simulink model "TopLevel_Turbofan_DT_healthy"  (R2025a)
settings: Solver=ode15s  StartTime=0.0  StopTime=500  MaxStep=0.01  RelTol=1e-3
undefined symbols (not defined in the file or in its folder): BPR_design, Eff_Fan_v1, Eff_HPC_v1, Eff_hpt_map, Eff_HPT_v1, Eff_LPC_v1, Eff_LPT_v1, eta_hpc_map, eta_lpc_map, eta_lpt_map, Fan_eta_data, Fan_PR_data, flow_vec_fan, norm_flow_hpt, norm_speed_hpt, PDM_Data, PR_hpc_map, PR_lpc_map, PR_lpt_map, speed_vec_fan, speed_vec_hpc, speed_vec_lpc, speed_vec_lpt, Torque_hpt_map, Wc_hpc_bp, Wc_lpc_bp, Wc_lpt_bp
libraries: fl_lib x10, nesl_utility x10, sdl_lib x2
settings Model: Creator=ramch  LastModifiedBy=ramch
settings DataIOCC: SaveFormat=StructureWithTime

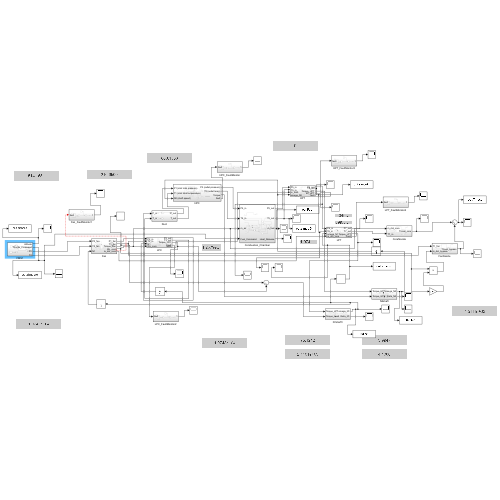
[thumbnail: Simulink's stored preview of the top-level diagram]
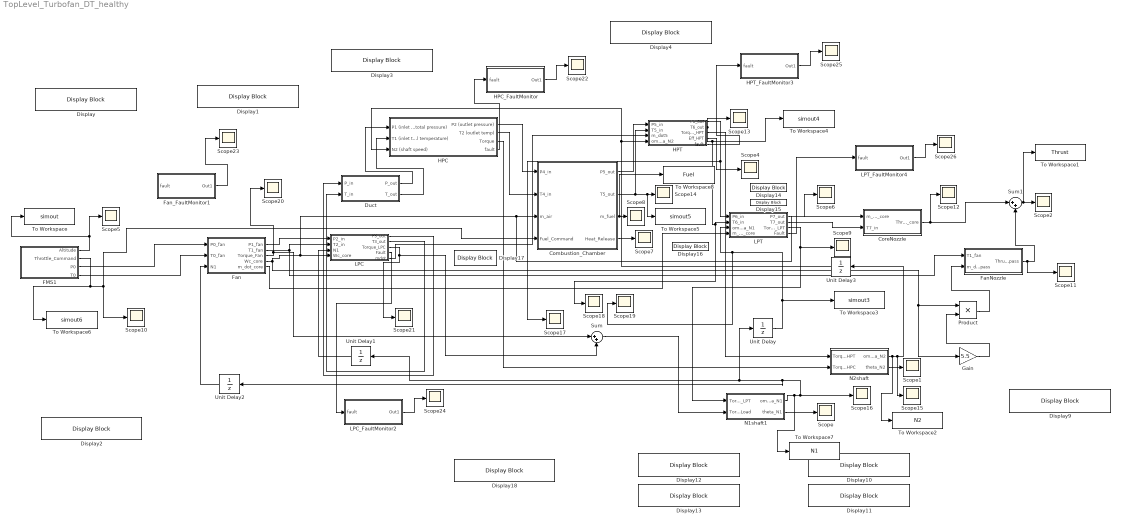
== system TopLevel_Turbofan_DT_healthy ==
  Combustion_Chamber : Subsystem
  CoreNozzle : Subsystem
  Display{,1..4,9..18} (15 alike) : DisplayBlock  LabelPosition=Hide  Transparency=1  GridColor=[0.502, 0.502, 0.502]
  Duct : Subsystem
  FMS1 : Subsystem
  Fan : Subsystem
  FanNozzle : Subsystem
  Fan_FaultMonitor1 : Subsystem
  Gain : Gain  Gain=5.5
  HPC : Subsystem
  HPC_FaultMonitor : Subsystem
  HPT : Subsystem
  HPT_FaultMonitor3 : Subsystem
  LPC : Subsystem
  LPC_FaultMonitor2 : Subsystem
  LPT : Subsystem
  LPT_FaultMonitor4 : Subsystem
  N1shaft1 : Subsystem
  N2shaft : Subsystem
  Product : Product
  Scope{,1..2,4..26} (26 alike) : Scope
      Scope settings: ActiveDisplayYMinimum=-1  ActiveDisplayYMaximum=1
      Scope1 settings: ActiveDisplayYMinimum=-1  ActiveDisplayYMaximum=1
      Scope10 settings: ActiveDisplayYMinimum=-0.45859345963387366  ActiveDisplayYMaximum=1.635778226221027  DataLoggingVariableName=ScopeData10
      Scope11 settings: ActiveDisplayYMinimum=-1  ActiveDisplayYMaximum=1  DataLoggingVariableName=ScopeData11
      Scope12 settings: ActiveDisplayYMinimum=-1  ActiveDisplayYMaximum=1  DataLoggingVariableName=ScopeData12
      Scope13 settings: ActiveDisplayYMinimum=-609.11434420859632  ActiveDisplayYMaximum=1781.0190470175871  DataLoggingVariableName=ScopeData13
      Scope14 settings: ActiveDisplayYMinimum=-1  ActiveDisplayYMaximum=1  DataLoggingVariableName=ScopeData14
      Scope15 settings: ActiveDisplayYMinimum=-1  ActiveDisplayYMaximum=1  DataLoggingVariableName=ScopeData15
      Scope16 settings: ActiveDisplayYMinimum=-4.3963021341582635  ActiveDisplayYMaximum=4.6281003390981308  DataLoggingVariableName=ScopeData16
      Scope17 settings: ActiveDisplayYMinimum=-2.2429279816897957E+23  ActiveDisplayYMaximum=2.0186351835208165E+24  DataLoggingVariableName=ScopeData17
      Scope18 settings: ActiveDisplayYMinimum=-513.71209028734575  ActiveDisplayYMaximum=1737.7811833983071  DataLoggingVariableName=ScopeData18
      Scope19 settings: ActiveDisplayYMinimum=-0.12499999999999997  ActiveDisplayYMaximum=1.125  DataLoggingVariableName=ScopeData19
      Scope2 settings: ActiveDisplayYMinimum=-1  ActiveDisplayYMaximum=1  DataLoggingVariableName=ScopeData2
      Scope20 settings: ActiveDisplayYMinimum=-3.6198875871994079E+21  ActiveDisplayYMaximum=5.5031192284267649E+20  DataLoggingVariableName=ScopeData20
      Scope21 settings: ActiveDisplayYMinimum=-0.23453341351778778  ActiveDisplayYMaximum=0.2421108240195578  DataLoggingVariableName=ScopeData21
      Scope22 settings: ActiveDisplayYMinimum=-609.11434420859632  ActiveDisplayYMaximum=1781.0190470175871  DataLoggingVariableName=ScopeData22
      Scope23 settings: ActiveDisplayYMinimum=-609.11434420859632  ActiveDisplayYMaximum=1781.0190470175871  DataLoggingVariableName=ScopeData23
      Scope24 settings: ActiveDisplayYMinimum=-609.11434420859632  ActiveDisplayYMaximum=1781.0190470175871  DataLoggingVariableName=ScopeData24
      Scope25 settings: ActiveDisplayYMinimum=-609.11434420859632  ActiveDisplayYMaximum=1781.0190470175871  DataLoggingVariableName=ScopeData25
      Scope26 settings: ActiveDisplayYMinimum=-609.11434420859632  ActiveDisplayYMaximum=1781.0190470175871  DataLoggingVariableName=ScopeData26
      Scope4 settings: ActiveDisplayYMinimum=-1.4197628335321743E+18  ActiveDisplayYMaximum=1.5775142594801933E+17  DataLoggingVariableName=ScopeData4
      Scope5 settings: ActiveDisplayYMinimum=-5201.9747686683695  ActiveDisplayYMaximum=12688.378863465885  DataLoggingVariableName=ScopeData5
      Scope6 settings: ActiveDisplayYMinimum=-1  ActiveDisplayYMaximum=1  DataLoggingVariableName=ScopeData6
      Scope7 settings: ActiveDisplayYMinimum=952444.62242727727  ActiveDisplayYMaximum=9.2631053030945715E+6  DataLoggingVariableName=ScopeData7
      Scope8 settings: ActiveDisplayYMinimum=-1  ActiveDisplayYMaximum=1  DataLoggingVariableName=ScopeData8
      Scope9 settings: ActiveDisplayYMinimum=-1  ActiveDisplayYMaximum=1  DataLoggingVariableName=ScopeData9
  Sum : Sum  Inputs=|++
  Sum1 : Sum  Inputs=|++
  To Workspace : ToWorkspace  VariableName=simout  SaveFormat=Timeseries  SampleTime=-1
  To Workspace1 : ToWorkspace  VariableName=Thrust  SaveFormat=Timeseries  SampleTime=-1
  To Workspace2 : ToWorkspace  VariableName=N2  SaveFormat=Timeseries  SampleTime=-1
  To Workspace3 : ToWorkspace  VariableName=simout3  SaveFormat=Timeseries  SampleTime=-1
  To Workspace4 : ToWorkspace  VariableName=simout4  SaveFormat=Timeseries  SampleTime=-1
  To Workspace5 : ToWorkspace  VariableName=simout5  SaveFormat=Timeseries  SampleTime=-1
  To Workspace6 : ToWorkspace  VariableName=simout6  SaveFormat=Timeseries  SampleTime=-1
  To Workspace7 : ToWorkspace  VariableName=N1  SaveFormat=Timeseries  SampleTime=-1
  To Workspace8 : ToWorkspace  VariableName=Fuel  SaveFormat=Timeseries  SampleTime=-1
  Unit Delay{,1..3} (4 alike) : UnitDelay  InitialCondition=1  SampleTime=-1  HasFrameUpgradeWarning=on
  wires:
  FMS1/3(P0) -> Fan/1(P0_fan)
  FMS1/4(T0) -> Fan/2(T0_fan)
  FMS1/2(Throttle_Command) -> To Workspace6/1, Combustion_Chamber/4(Fuel_Command), Scope10/1
  Fan/1(" P1_fan") -> LPC/1(P2_in)
  Fan/2(T1_fan) -> LPC/2(T2_in), FanNozzle/1(T1_fan)
  Fan/4(Wc_core) -> Gain/1, Product/1, CoreNozzle/1(m_dot_core), Combustion_Chamber/3(m_air), LPC/4(Wc_core)
  LPC/1(P3_out) -> Duct/1(P_in)
  Duct/1(P_out) -> HPC/1(P1 (inlet total pressure))
  Duct/2(T_out) -> HPC/2("T1 (inlet total temperature) ")
  HPC/1(P2 (outlet pressure)) -> Combustion_Chamber/1(P4_in)
  HPC/2(T2 (outlet temp)) -> Combustion_Chamber/2(T4_in)
  Combustion_Chamber/1(P5_out) -> HPT/1(P5_in)
  Combustion_Chamber/2(T5_out) -> To Workspace5/1, Scope14/1, HPT/2(T5_in)
  HPT/1(P6_out) -> LPT/1(P6_in), Scope17/1
  HPT/2(T6_out) -> To Workspace4/1, Scope18/1, LPT/2(T6_in), Scope13/1
  LPT/3(Torque_LPT) -> N1shaft1/1(Torque_LPT), Scope9/1
  Sum/1 -> N1shaft1/2(Torque_Load)
  LPC/3(Torque_LPC) -> Scope21/1, Sum/2
  Fan/3(Torque_Fan) -> Scope20/1, Sum/1
  HPC/3(Torque) -> N2shaft/2(Torque_HPC)
  HPT/3(Torque_HPT) -> N2shaft/1(Torque_HPT)
  N2shaft/1(omega_N2) -> To Workspace2/1, Scope15/1, Unit Delay3/1
  LPT/2(T7_out) -> CoreNozzle/2(T7_in)
  Product/1 -> FanNozzle/2(m_dot_bypass)
  Gain/1 -> Product/2
  FanNozzle/1(Thrust_bypass) -> Scope11/1, Sum1/2
  CoreNozzle/1(Thrust_core) -> Scope12/1, Sum1/1
  Sum1/1 -> To Workspace1/1, Scope2/1
  N2shaft/2(theta_N2) -> Scope1/1
  LPC/2(T3_out) -> Duct/2(T_in)
  FMS1/1(Altitude) -> To Workspace/1, Scope5/1
  HPT/4(Eff_HPT) -> Scope4/1
  LPT/1(P7_out) -> Scope6/1
  Combustion_Chamber/3(m_fuel) -> To Workspace8/1, Scope8/1
  Combustion_Chamber/4(Heat_Release) -> Scope7/1
  N1shaft1/2(theta_N1) -> Scope/1
  N1shaft1/1(omega_N1) -> To Workspace7/1, Unit Delay/1, Unit Delay1/1, Unit Delay2/1, Scope16/1
  Unit Delay/1 -> Scope19/1, LPT/3(omega_N1), To Workspace3/1
  Unit Delay2/1 -> Fan/3(N1)
  Unit Delay1/1 -> LPC/3(N1)
  HPC_FaultMonitor/1(Out1) -> Scope22/1
  HPC/4(fault) -> HPC_FaultMonitor/1(fault)
  Fan_FaultMonitor1/1(Out1) -> Scope23/1
  LPC_FaultMonitor2/1(Out1) -> Scope24/1
  HPT_FaultMonitor3/1(Out1) -> Scope25/1
  LPT_FaultMonitor4/1(Out1) -> Scope26/1
  ? -> Fan_FaultMonitor1/1(fault)
  LPC/4(Fault) -> LPC_FaultMonitor2/1(fault)
  HPT/5(fault) -> HPT_FaultMonitor3/1(fault)
  LPT/4(Fault) -> LPT_FaultMonitor4/1(fault)
  Unit Delay3/1 -> HPT/4(omega_N2), HPC/3(N2 (shaft speed))
  LPC/5(mdot) -> HPT/3(m_dot5)
  Fan/5(m_dot_core) -> LPT/4(m_dot_core)

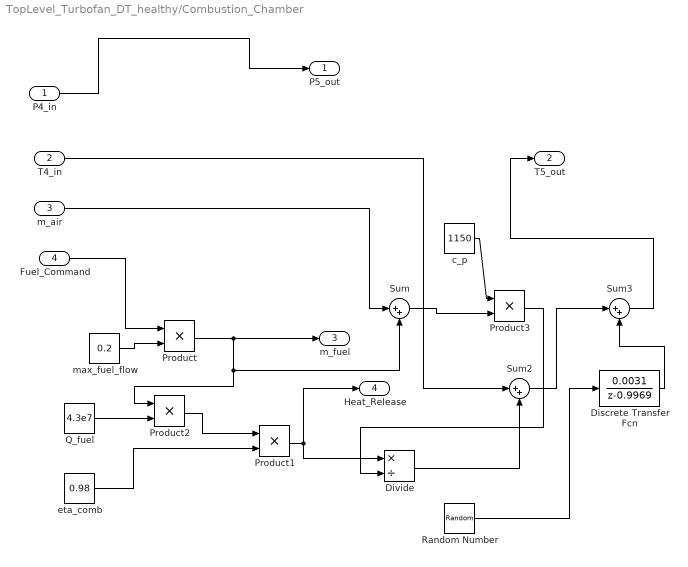
== system TopLevel_Turbofan_DT_healthy/Combustion_Chamber ==
  P4_in : Inport
  T4_in : Inport  Port=2
  m_air : Inport  Port=3
  Fuel_Command : Inport  Port=4
  Discrete Transfer Fcn : DiscreteTransferFcn  Numerator=0.0031  Denominator=1 -0.9969  InitialStates=0.001
  Divide : Product  Inputs=*/
  Product{,1..3} (4 alike) : Product
  Q_fuel : Constant  Value=4.3e7
  Random Number : RandomNumber  Variance=0.5  SampleTime=0.001
  Sum : Sum  Inputs=|++
  Sum2 : Sum  Inputs=|++
  Sum3 : Sum  Inputs=|++
  c_p : Constant  Value=1150
  eta_comb : Constant  Value=0.98
  max_fuel_flow : Constant  Value=0.2
  P5_out : Outport
  T5_out : Outport  Port=2
  m_fuel : Outport  Port=3
  Heat_Release : Outport  Port=4
  wires:
  Discrete Transfer Fcn/1 -> Sum3/2
  Sum2/1 -> Sum3/1
  Sum3/1 -> T5_out/1
  Random Number/1 -> Discrete Transfer Fcn/1
  Divide/1 -> Sum2/2
  T4_in/1 -> Sum2/1
  Product3/1 -> Divide/2
  c_p/1 -> Product3/1
  Sum/1 -> Product3/2
  P4_in/1 -> P5_out/1
  m_air/1 -> Sum/1
  Product2/1 -> Product1/1
  Product/1 -> m_fuel/1, Sum/2, Product2/1
  Product1/1 -> Divide/1, Heat_Release/1
  eta_comb/1 -> Product1/2
  Q_fuel/1 -> Product2/2
  max_fuel_flow/1 -> Product/2
  Fuel_Command/1 -> Product/1

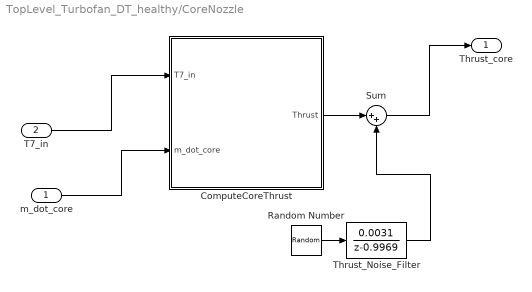
== system TopLevel_Turbofan_DT_healthy/CoreNozzle ==
  m_dot_core : Inport
  T7_in : Inport  Port=2
  ComputeCoreThrust : MATLAB Function  TreatAsAtomicUnit=on
  Random Number : RandomNumber  Variance=500  SampleTime=0.001
  Sum : Sum  Inputs=|++
  Thrust_Noise_Filter : DiscreteTransferFcn  Numerator=0.0031  Denominator=1 -0.9969  InitialStates=0.001
  Thrust_core : Outport
  wires:
  Sum/1 -> Thrust_core/1
  T7_in/1 -> ComputeCoreThrust/1(T7_in)
  Random Number/1 -> Thrust_Noise_Filter/1
  m_dot_core/1 -> ComputeCoreThrust/2(m_dot_core)
  ComputeCoreThrust/1(Thrust) -> Sum/1
  Thrust_Noise_Filter/1 -> Sum/2

== system TopLevel_Turbofan_DT_healthy/Duct ==
  P_in : Inport
  T_in : Inport  Port=2
  Gain : Gain  Gain=0.98
  P_out : Outport
  T_out : Outport  Port=2
  wires:
  Gain/1 -> P_out/1
  T_in/1 -> T_out/1
  P_in/1 -> Gain/1

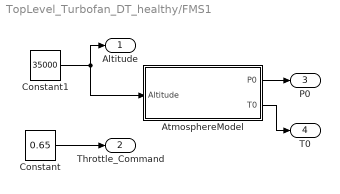
== system TopLevel_Turbofan_DT_healthy/FMS1 ==
  AtmosphereModel : MATLAB Function  TreatAsAtomicUnit=on
  Constant : Constant  Value=0.65
  Constant1 : Constant  Value=35000
  Altitude : Outport
  Throttle_Command : Outport  Port=2
  P0 : Outport  Port=3
  T0 : Outport  Port=4
  wires:
  AtmosphereModel/1(P0) -> P0/1
  AtmosphereModel/2(T0) -> T0/1
  Constant1/1 -> AtmosphereModel/1(Altitude), Altitude/1
  Constant/1 -> Throttle_Command/1

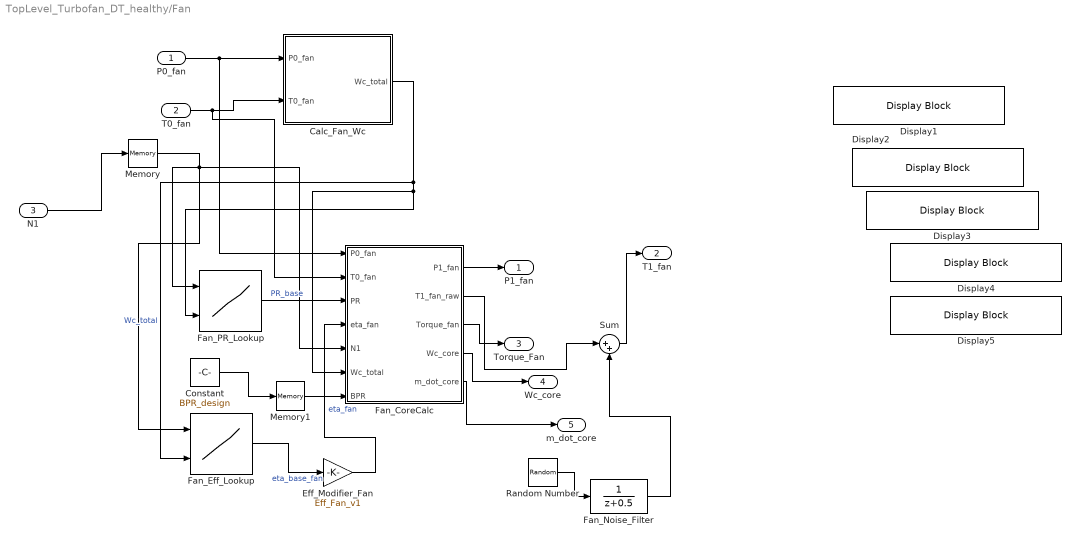
== system TopLevel_Turbofan_DT_healthy/Fan ==
  P0_fan : Inport
  T0_fan : Inport  Port=2
  N1 : Inport  Port=3
  Calc_Fan_Wc : MATLAB Function  TreatAsAtomicUnit=on
  Constant : Constant  Value=BPR_design
  Display{1..5} (5 alike) : DisplayBlock  LabelPosition=Hide  Transparency=1  GridColor=[0.502, 0.502, 0.502]
  Eff_Modifier_Fan : Gain  Gain=Eff_Fan_v1
  Fan_CoreCalc : MATLAB Function  TreatAsAtomicUnit=on
  Fan_Eff_Lookup : Lookup_n-D  BreakpointsForDimension1=speed_vec_fan  BreakpointsForDimension2=flow_vec_fan  Table=Fan_eta_data  ExtrapMethod=Clip  InternalRulePriority=Speed  RndMeth=Simplest
      settings: InputPortMap=u0,u1
  Fan_Noise_Filter : DiscreteTransferFcn
  Fan_PR_Lookup : Lookup_n-D  BreakpointsForDimension1=speed_vec_fan  BreakpointsForDimension2=flow_vec_fan  Table=Fan_PR_data  ExtrapMethod=Clip  InternalRulePriority=Speed  RndMeth=Simplest
      settings: InputPortMap=u0,u1
  Memory : Memory
  Memory1 : Memory
  Random Number : RandomNumber  Variance=(0.5)  SampleTime=0.001
  Sum : Sum  Inputs=|++
  " P1_fan" : Outport
  T1_fan : Outport  Port=2
  Torque_Fan : Outport  Port=3
  Wc_core : Outport  Port=4
  m_dot_core : Outport  Port=5
  wires:
  Random Number/1 -> Fan_Noise_Filter/1
  Fan_Noise_Filter/1 -> Sum/2
  Fan_CoreCalc/2(T1_fan_raw) -> Sum/1
  Sum/1 -> T1_fan/1
  Fan_CoreCalc/1(P1_fan) -> " P1_fan"/1
  Fan_CoreCalc/3(Torque_fan) -> Torque_Fan/1
  Fan_CoreCalc/4(Wc_core) -> Wc_core/1
  Fan_PR_Lookup/1 -> Fan_CoreCalc/3(PR)  "PR_base"
  Eff_Modifier_Fan/1 -> Fan_CoreCalc/4(eta_fan)  "eta_fan"
  Fan_Eff_Lookup/1 -> Eff_Modifier_Fan/1  "eta_base_fan"
  Calc_Fan_Wc/1(Wc_total) -> Fan_Eff_Lookup/2, Fan_PR_Lookup/2, Fan_CoreCalc/6(Wc_total)  "Wc_total"
  T0_fan/1 -> Calc_Fan_Wc/2(T0_fan), Fan_CoreCalc/2(T0_fan)
  P0_fan/1 -> Calc_Fan_Wc/1(P0_fan), Fan_CoreCalc/1(P0_fan)
  Memory1/1 -> Fan_CoreCalc/7(BPR)
  Memory/1 -> Fan_Eff_Lookup/1, Fan_PR_Lookup/1, Fan_CoreCalc/5(N1)
  Constant/1 -> Memory1/1
  N1/1 -> Memory/1
  Fan_CoreCalc/5(m_dot_core) -> m_dot_core/1

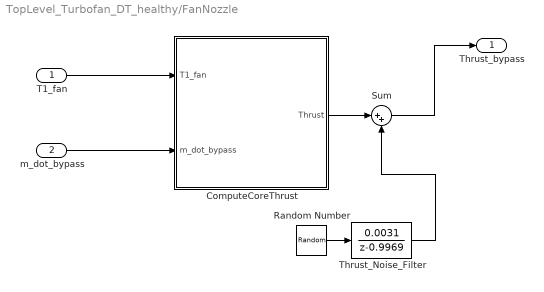
== system TopLevel_Turbofan_DT_healthy/FanNozzle ==
  T1_fan : Inport
  m_dot_bypass : Inport  Port=2
  ComputeCoreThrust : MATLAB Function  TreatAsAtomicUnit=on
  Random Number : RandomNumber  Variance=200  SampleTime=0.001
  Sum : Sum  Inputs=|++
  Thrust_Noise_Filter : DiscreteTransferFcn  Numerator=0.0031  Denominator=1 -0.9969  InitialStates=0.001
  Thrust_bypass : Outport
  wires:
  T1_fan/1 -> ComputeCoreThrust/1(T1_fan)
  Random Number/1 -> Thrust_Noise_Filter/1
  Sum/1 -> Thrust_bypass/1
  Thrust_Noise_Filter/1 -> Sum/2
  ComputeCoreThrust/1(Thrust) -> Sum/1
  m_dot_bypass/1 -> ComputeCoreThrust/2(m_dot_bypass)

== system TopLevel_Turbofan_DT_healthy/Fan_FaultMonitor1 ==
  fault : Inport
  Constant : Constant  Value=0.95
  Constant1 : Constant  Value=0.05
  Relational Operator : RelationalOperator  Operator=>  OutDataTypeStr=boolean  RndMeth=Simplest  InputSameDT=off
  Subtract : Sum  Inputs=+-
  Out1 : Outport
  wires:
  Constant/1 -> Subtract/1
  fault/1 -> Subtract/2
  Subtract/1 -> Relational Operator/2
  Constant1/1 -> Relational Operator/1
  Relational Operator/1 -> Out1/1

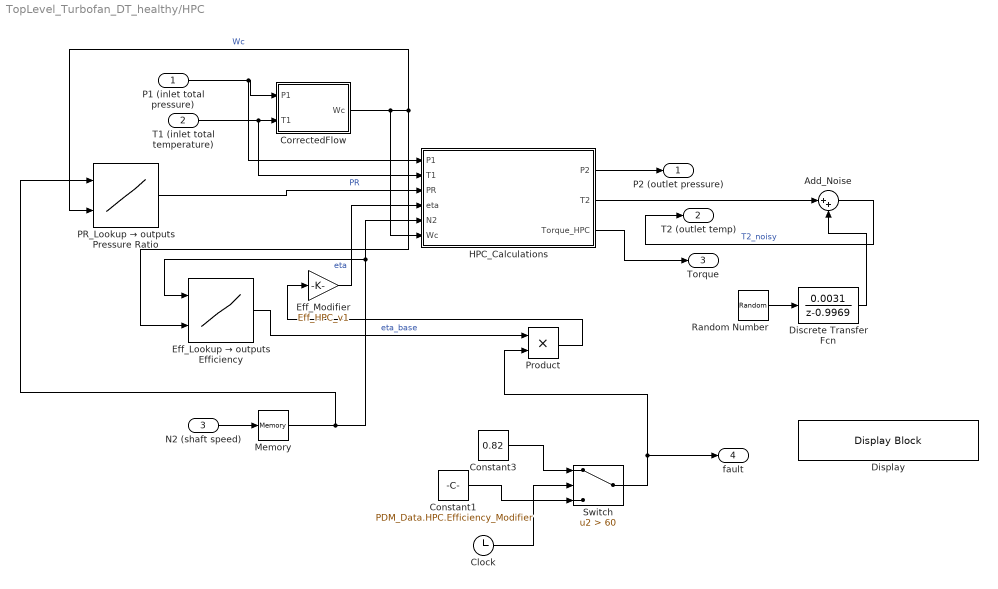
== system TopLevel_Turbofan_DT_healthy/HPC ==
  P1 (inlet total pressure) : Inport
  "T1 (inlet total temperature) " : Inport  Port=2
  N2 (shaft speed) : Inport  Port=3
  Add_Noise : Sum  Inputs=|++
  Clock : Clock
  Constant1 : Constant  Value=PDM_Data.HPC.Efficiency_Modifier
  Constant3 : Constant  Value=0.82
  CorrectedFlow : MATLAB Function  TreatAsAtomicUnit=on
  Discrete Transfer Fcn : DiscreteTransferFcn  Numerator=0.0031  Denominator=1 -0.9969  InitialStates=0.001
  Display : DisplayBlock  LabelPosition=Hide  Transparency=1  GridColor=[0.502, 0.502, 0.502]
  Eff_Lookup → outputs Efficiency : Lookup_n-D  BreakpointsForDimension1=speed_vec_hpc  BreakpointsForDimension2=Wc_hpc_bp  Table=eta_hpc_map  InternalRulePriority=Speed  RndMeth=Simplest
      settings: InputPortMap=u0,u1
  Eff_Modifier : Gain  Gain=Eff_HPC_v1
  HPC_Calculations : MATLAB Function  TreatAsAtomicUnit=on
  Memory : Memory
  PR_Lookup → outputs Pressure Ratio : Lookup_n-D  BreakpointsForDimension1=speed_vec_hpc  BreakpointsForDimension2=Wc_hpc_bp  Table=PR_hpc_map  InternalRulePriority=Speed  RndMeth=Simplest
      settings: InputPortMap=u0,u1
  Product : Product
  Random Number : RandomNumber  Variance=(0.5)  SampleTime=0.001
  Switch : Switch  Criteria=u2 > Threshold  Threshold=60  SaturateOnIntegerOverflow=off  InputSameDT=off
  P2 (outlet pressure) : Outport
  T2 (outlet temp) : Outport  Port=2
  Torque : Outport  Port=3
  fault : Outport  Port=4
  wires:
  Random Number/1 -> Discrete Transfer Fcn/1
  Discrete Transfer Fcn/1 -> Add_Noise/2
  Add_Noise/1 -> T2 (outlet temp)/1  "T2_noisy"
  Eff_Modifier/1 -> HPC_Calculations/4(eta)  "eta"
  CorrectedFlow/1(Wc) -> Eff_Lookup → outputs Efficiency/2, PR_Lookup → outputs Pressure Ratio/2, HPC_Calculations/6(Wc)  "Wc"
  "T1 (inlet total temperature) "/1 -> CorrectedFlow/2(T1), HPC_Calculations/2(T1)
  P1 (inlet total pressure)/1 -> CorrectedFlow/1(P1), HPC_Calculations/1(P1)
  N2 (shaft speed)/1 -> Memory/1
  Eff_Lookup → outputs Efficiency/1 -> Product/1  "eta_base"
  PR_Lookup → outputs Pressure Ratio/1 -> HPC_Calculations/3(PR)  "PR"
  HPC_Calculations/3(Torque_HPC) -> Torque/1
  HPC_Calculations/2(T2) -> Add_Noise/1
  HPC_Calculations/1(P2) -> P2 (outlet pressure)/1
  Memory/1 -> HPC_Calculations/5(N2), Eff_Lookup → outputs Efficiency/1, PR_Lookup → outputs Pressure Ratio/1
  Product/1 -> Eff_Modifier/1
  Constant3/1 -> Switch/1
  Switch/1 -> Product/2, fault/1
  Clock/1 -> Switch/2
  Constant1/1 -> Switch/3

== system TopLevel_Turbofan_DT_healthy/HPC_FaultMonitor ==
  fault : Inport
  Constant : Constant  Value=0.92
  Constant1 : Constant  Value=0.05
  Relational Operator : RelationalOperator  Operator=>  OutDataTypeStr=boolean  RndMeth=Simplest  InputSameDT=off
  Subtract : Sum  Inputs=+-
  Out1 : Outport
  wires:
  Constant/1 -> Subtract/1
  fault/1 -> Subtract/2
  Subtract/1 -> Relational Operator/2
  Constant1/1 -> Relational Operator/1
  Relational Operator/1 -> Out1/1

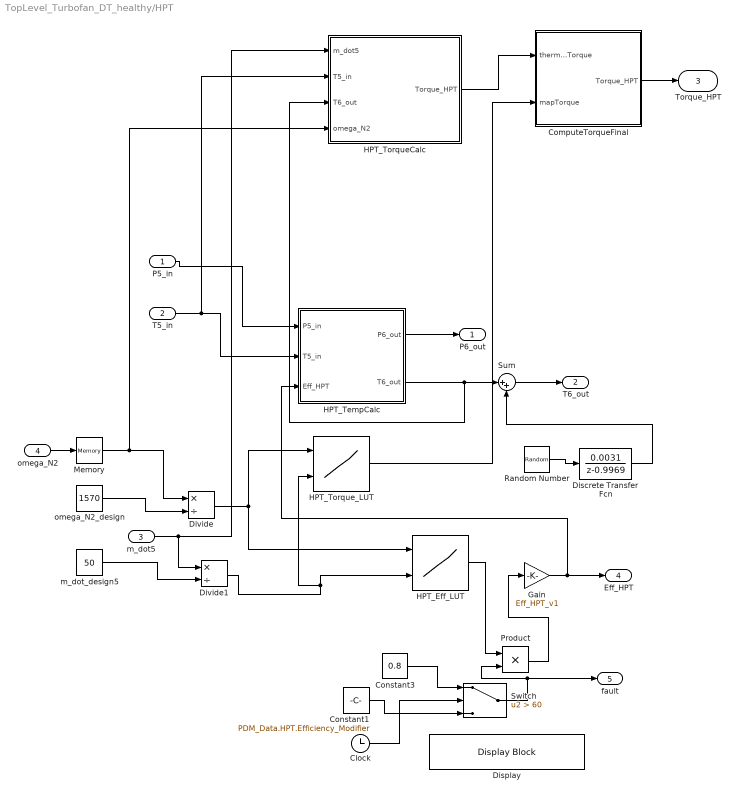
== system TopLevel_Turbofan_DT_healthy/HPT ==
  P5_in : Inport
  T5_in : Inport  Port=2
  m_dot5 : Inport  Port=3
  omega_N2 : Inport  Port=4
  Clock : Clock
  ComputeTorqueFinal : MATLAB Function  TreatAsAtomicUnit=on
  Constant1 : Constant  Value=PDM_Data.HPT.Efficiency_Modifier
  Constant3 : Constant  Value=0.8
  Discrete Transfer Fcn : DiscreteTransferFcn  Numerator=0.0031  Denominator=1 -0.9969  InitialStates=0.001
  Display : DisplayBlock  LabelPosition=Hide  Transparency=1  GridColor=[0.502, 0.502, 0.502]
  Divide : Product  Inputs=*/
  Divide1 : Product  Inputs=*/
  Gain : Gain  Gain=Eff_HPT_v1
  HPT_Eff_LUT : Lookup_n-D  BreakpointsForDimension1=norm_speed_hpt  BreakpointsForDimension2=norm_flow_hpt  Table=Eff_hpt_map  InternalRulePriority=Speed  RndMeth=Simplest
      settings: InputPortMap=u0,u1
  HPT_TempCalc : MATLAB Function  TreatAsAtomicUnit=on
  HPT_TorqueCalc : MATLAB Function  TreatAsAtomicUnit=on
  HPT_Torque_LUT : Lookup_n-D  BreakpointsForDimension1=norm_speed_hpt  BreakpointsForDimension2=norm_flow_hpt  Table=Torque_hpt_map  InternalRulePriority=Speed  RndMeth=Simplest
      settings: InputPortMap=u0,u1
  Memory : Memory
  Product : Product
  Random Number : RandomNumber  Variance=0.5  SampleTime=0.1
  Sum : Sum  Inputs=|++
  Switch : Switch  Criteria=u2 > Threshold  Threshold=60  SaturateOnIntegerOverflow=off  InputSameDT=off
  m_dot_design5 : Constant  Value=50
  omega_N2_design : Constant  Value=1570
  P6_out : Outport
  T6_out : Outport  Port=2
  Torque_HPT : Outport  Port=3
  Eff_HPT : Outport  Port=4
  fault : Outport  Port=5
  wires:
  HPT_Torque_LUT/1 -> ComputeTorqueFinal/2(mapTorque)
  HPT_TorqueCalc/1(Torque_HPT) -> ComputeTorqueFinal/1(thermoTorque)
  ComputeTorqueFinal/1(Torque_HPT) -> Torque_HPT/1
  Random Number/1 -> Discrete Transfer Fcn/1
  Sum/1 -> T6_out/1
  Discrete Transfer Fcn/1 -> Sum/2
  HPT_TempCalc/2(T6_out) -> Sum/1, HPT_TorqueCalc/3(T6_out)
  HPT_TempCalc/1(P6_out) -> P6_out/1
  T5_in/1 -> HPT_TempCalc/2(T5_in), HPT_TorqueCalc/2(T5_in)
  Gain/1 -> Eff_HPT/1, HPT_TempCalc/3(Eff_HPT)
  HPT_Eff_LUT/1 -> Product/1
  P5_in/1 -> HPT_TempCalc/1(P5_in)
  Divide1/1 -> HPT_Eff_LUT/2, HPT_Torque_LUT/2
  Divide/1 -> HPT_Torque_LUT/1, HPT_Eff_LUT/1
  omega_N2/1 -> Memory/1
  omega_N2_design/1 -> Divide/2
  m_dot5/1 -> Divide1/1, HPT_TorqueCalc/1(m_dot5)
  m_dot_design5/1 -> Divide1/2
  Memory/1 -> Divide/1, HPT_TorqueCalc/4(omega_N2)
  Product/1 -> Gain/1
  Constant3/1 -> Switch/1
  Switch/1 -> fault/1, Product/2
  Clock/1 -> Switch/2
  Constant1/1 -> Switch/3

== system TopLevel_Turbofan_DT_healthy/HPT_FaultMonitor3 ==
  fault : Inport
  Constant : Constant  Value=0.97
  Constant1 : Constant  Value=0.05
  Relational Operator : RelationalOperator  Operator=>  OutDataTypeStr=boolean  RndMeth=Simplest  InputSameDT=off
  Subtract : Sum  Inputs=+-
  Out1 : Outport
  wires:
  Constant/1 -> Subtract/1
  fault/1 -> Subtract/2
  Subtract/1 -> Relational Operator/2
  Constant1/1 -> Relational Operator/1
  Relational Operator/1 -> Out1/1

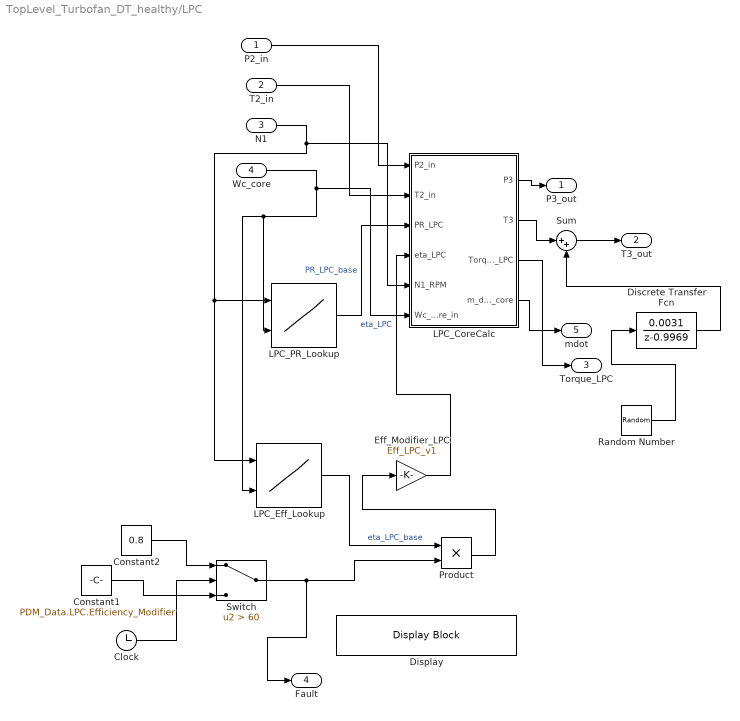
== system TopLevel_Turbofan_DT_healthy/LPC ==
  P2_in : Inport
  T2_in : Inport  Port=2
  N1 : Inport  Port=3
  Wc_core : Inport  Port=4
  Clock : Clock
  Constant1 : Constant  Value=PDM_Data.LPC.Efficiency_Modifier
  Constant2 : Constant  Value=0.8
  Discrete Transfer Fcn : DiscreteTransferFcn  Numerator=0.0031  Denominator=1 -0.9969  InitialStates=0.001
  Display : DisplayBlock  LabelPosition=Hide  Transparency=1  GridColor=[0.502, 0.502, 0.502]
  Eff_Modifier_LPC : Gain  Gain=Eff_LPC_v1
  LPC_CoreCalc : MATLAB Function  TreatAsAtomicUnit=on
  LPC_Eff_Lookup : Lookup_n-D  BreakpointsForDimension1=speed_vec_lpc  BreakpointsForDimension2=Wc_lpc_bp  Table=eta_lpc_map  ExtrapMethod=Clip  InternalRulePriority=Speed  RndMeth=Simplest
      settings: InputPortMap=u0,u1
  LPC_PR_Lookup : Lookup_n-D  BreakpointsForDimension1=speed_vec_lpc  BreakpointsForDimension2=Wc_lpc_bp  Table=PR_lpc_map  ExtrapMethod=Clip  InternalRulePriority=Speed  RndMeth=Simplest
      settings: InputPortMap=u0,u1
  Product : Product
  Random Number : RandomNumber  Variance=(0.5)  SampleTime=0.001
  Sum : Sum  Inputs=|++
  Switch : Switch  Criteria=u2 > Threshold  Threshold=60  SaturateOnIntegerOverflow=off  InputSameDT=off
  P3_out : Outport
  T3_out : Outport  Port=2
  Torque_LPC : Outport  Port=3
  Fault : Outport  Port=4
  mdot : Outport  Port=5
  wires:
  Discrete Transfer Fcn/1 -> Sum/2
  Random Number/1 -> Discrete Transfer Fcn/1
  Sum/1 -> T3_out/1
  LPC_CoreCalc/2(T3) -> Sum/1
  LPC_CoreCalc/3(Torque_LPC) -> Torque_LPC/1
  LPC_CoreCalc/1(P3) -> P3_out/1
  Eff_Modifier_LPC/1 -> LPC_CoreCalc/4(eta_LPC)  "eta_LPC"
  LPC_PR_Lookup/1 -> LPC_CoreCalc/3(PR_LPC)  "PR_LPC_base"
  T2_in/1 -> LPC_CoreCalc/2(T2_in)
  P2_in/1 -> LPC_CoreCalc/1(P2_in)
  LPC_Eff_Lookup/1 -> Product/1  "eta_LPC_base"
  Wc_core/1 -> LPC_PR_Lookup/2, LPC_Eff_Lookup/2, LPC_CoreCalc/6(Wc_core_in)
  N1/1 -> LPC_PR_Lookup/1, LPC_Eff_Lookup/1, LPC_CoreCalc/5(N1_RPM)
  Product/1 -> Eff_Modifier_LPC/1
  Constant2/1 -> Switch/1
  Switch/1 -> Fault/1, Product/2
  LPC_CoreCalc/4(m_dot_core) -> mdot/1
  Clock/1 -> Switch/2
  Constant1/1 -> Switch/3

== system TopLevel_Turbofan_DT_healthy/LPC_FaultMonitor2 ==
  fault : Inport
  Constant : Constant  Value=0.9
  Constant1 : Constant  Value=0.05
  Relational Operator : RelationalOperator  Operator=>  OutDataTypeStr=boolean  RndMeth=Simplest  InputSameDT=off
  Subtract : Sum  Inputs=+-
  Out1 : Outport
  wires:
  Constant/1 -> Subtract/1
  fault/1 -> Subtract/2
  Subtract/1 -> Relational Operator/2
  Constant1/1 -> Relational Operator/1
  Relational Operator/1 -> Out1/1

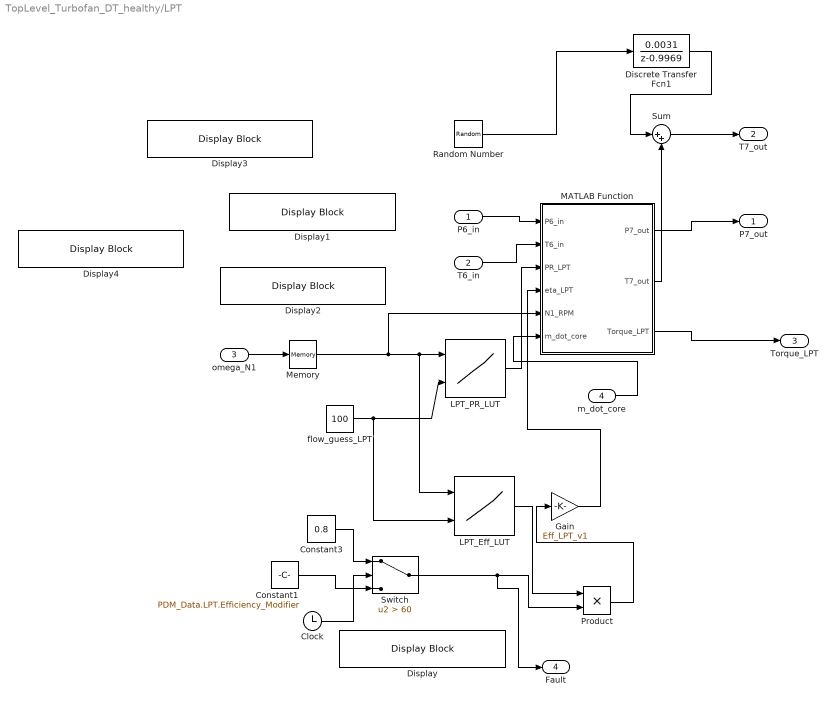
== system TopLevel_Turbofan_DT_healthy/LPT ==
  P6_in : Inport
  T6_in : Inport  Port=2
  omega_N1 : Inport  Port=3
  m_dot_core : Inport  Port=4
  Clock : Clock
  Constant1 : Constant  Value=PDM_Data.LPT.Efficiency_Modifier
  Constant3 : Constant  Value=0.8
  Discrete Transfer Fcn1 : DiscreteTransferFcn  Numerator=0.0031  Denominator=1 -0.9969  InitialStates=0.001
  Display{,1..4} (5 alike) : DisplayBlock  LabelPosition=Hide  Transparency=1  GridColor=[0.502, 0.502, 0.502]
  Gain : Gain  Gain=Eff_LPT_v1
  LPT_Eff_LUT : Lookup_n-D  BreakpointsForDimension1=speed_vec_lpt  BreakpointsForDimension2=Wc_lpt_bp  Table=eta_lpt_map  ExtrapMethod=Clip  InternalRulePriority=Speed  RndMeth=Simplest
      settings: InputPortMap=u0,u1
  LPT_PR_LUT : Lookup_n-D  BreakpointsForDimension1=speed_vec_lpt  BreakpointsForDimension2=Wc_lpt_bp  Table=PR_lpt_map  ExtrapMethod=Clip  InternalRulePriority=Speed  RndMeth=Simplest
      settings: InputPortMap=u0,u1
  MATLAB Function : MATLAB Function  TreatAsAtomicUnit=on
  Memory : Memory
  Product : Product
  Random Number : RandomNumber  Variance=0.5  SampleTime=0.001
  Sum : Sum  Inputs=|++
  Switch : Switch  Criteria=u2 > Threshold  Threshold=60  SaturateOnIntegerOverflow=off  InputSameDT=off
  flow_guess_LPT : Constant  Value=100
  P7_out : Outport
  T7_out : Outport  Port=2
  Torque_LPT : Outport  Port=3
  Fault : Outport  Port=4
  wires:
  MATLAB Function/2(T7_out) -> Sum/2
  Gain/1 -> MATLAB Function/4(eta_LPT)
  LPT_Eff_LUT/1 -> Product/1
  MATLAB Function/1(P7_out) -> P7_out/1
  MATLAB Function/3(Torque_LPT) -> Torque_LPT/1
  flow_guess_LPT/1 -> LPT_Eff_LUT/2, LPT_PR_LUT/2
  omega_N1/1 -> Memory/1
  T6_in/1 -> MATLAB Function/2(T6_in)
  Sum/1 -> T7_out/1
  Discrete Transfer Fcn1/1 -> Sum/1
  Random Number/1 -> Discrete Transfer Fcn1/1
  LPT_PR_LUT/1 -> MATLAB Function/3(PR_LPT)
  P6_in/1 -> MATLAB Function/1(P6_in)
  Memory/1 -> LPT_PR_LUT/1, LPT_Eff_LUT/1, MATLAB Function/5(N1_RPM)
  Product/1 -> Gain/1
  Constant3/1 -> Switch/1
  Switch/1 -> Fault/1, Product/2
  Constant1/1 -> Switch/3
  Clock/1 -> Switch/2
  m_dot_core/1 -> MATLAB Function/6(m_dot_core)

== system TopLevel_Turbofan_DT_healthy/LPT_FaultMonitor4 ==
  fault : Inport
  Constant : Constant  Value=0.96
  Constant1 : Constant  Value=0.05
  Relational Operator : RelationalOperator  Operator=>  OutDataTypeStr=boolean  RndMeth=Simplest  InputSameDT=off
  Subtract : Sum  Inputs=+-
  Out1 : Outport
  wires:
  Constant/1 -> Subtract/1
  fault/1 -> Subtract/2
  Subtract/1 -> Relational Operator/2
  Constant1/1 -> Relational Operator/1
  Relational Operator/1 -> Out1/1

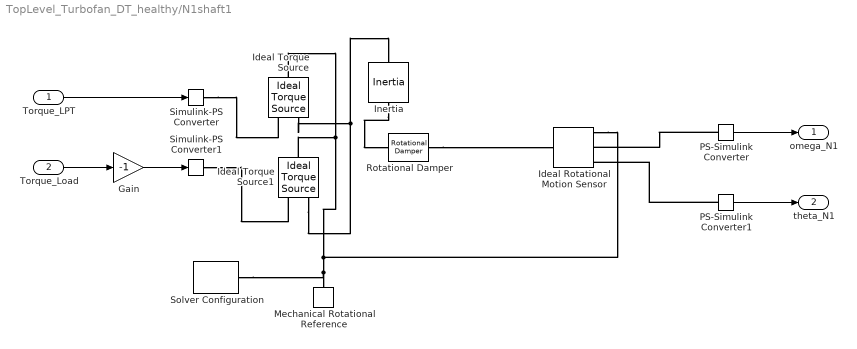
== system TopLevel_Turbofan_DT_healthy/N1shaft1 ==
  Torque_LPT : Inport
  Torque_Load : Inport  Port=2
  Gain : Gain  Gain=-1
  Ideal Rotational Motion Sensor : fl_lib/Mechanical/Mechanical Sensors/Ideal Rotational Motion Sensor  reference=foundation.enum.MeasurementReference.difference  acceleration_port=false  velocity_port=true  position_port=true  wrap_angle=false  offset=0 rad
  Ideal Torque Source : fl_lib/Mechanical/Mechanical Sources/Ideal Torque Source
  Ideal Torque Source1 : fl_lib/Mechanical/Mechanical Sources/Ideal Torque Source
  Inertia : fl_lib/Mechanical/Rotational Elements/Inertia  inertia=100 kg*m^2  num_ports=foundation.enum.numPorts2.two  w_specify=off  w_priority=High  w=52.36 rad/s  w_nominal_specify=off  w_nominal_value=1  w_nominal_unit=rad/s  t_specify=off  t_priority=None  t=0 N*m  t_nominal_specify=off  t_nominal_value=1  t_nominal_unit=N*m
      settings: InternalSimscapePortConfiguration="{\"Bottom\":[],\"Left\":[{\"id\":\"I\",\"label\":\"\",\"type\":\"foundation.mechanical.rotational.rotational\"}],\"Right\":[{\"id\":\"J\",\"label\":\"\",\"type\":\"foundation.mechanical.rotational.rotational\"}],\"Top\":[]}"
  Mechanical Rotational Reference : fl_lib/Mechanical/Rotational Elements/Mechanical Rotational Reference
  PS-Simulink Converter : nesl_utility/PS-Simulink Converter  PhysicalDomain=network_engine_domain  SubClassName=ps_output  LeftPortType=input  RightPortType=output  PseudoPeriodic=off  Frequencies=[]  VectorFormat=inherit  Unit=rad/s  AffineConversion=off
  PS-Simulink Converter1 : nesl_utility/PS-Simulink Converter  PhysicalDomain=network_engine_domain  SubClassName=ps_output  LeftPortType=input  RightPortType=output  PseudoPeriodic=off  Frequencies=[]  VectorFormat=inherit  Unit=rad  AffineConversion=off
  Rotational Damper : sdl_lib/Couplings & Drives/Springs & Dampers/Rotational Damper  D=10 N*m*s/rad  thermal_port=simscape.enum.thermaleffects.omit  thermal_mass=50 kJ/K  temperature_specify=off  temperature_priority=High  temperature=300 K  temperature_nominal_specify=off  temperature_nominal_value=1  temperature_nominal_unit=K
  Simulink-PS Converter : nesl_utility/Simulink-PS Converter  PhysicalDomain=network_engine_domain  SubClassName=ps_input  LeftPortType=input  RightPortType=output  PseudoPeriodic=off  Frequencies=[]  NoiseDistribution=none  NoiseParameters=[]  Unit=N*m  AffineConversion=off  FilteringAndDerivatives=provide  SimscapeFilterOrder=1  InputFilterTimeConstant=0.001  UdotUserProvided=0
  Simulink-PS Converter1 : nesl_utility/Simulink-PS Converter  PhysicalDomain=network_engine_domain  SubClassName=ps_input  LeftPortType=input  RightPortType=output  PseudoPeriodic=off  Frequencies=[]  NoiseDistribution=none  NoiseParameters=[]  Unit=N*m  AffineConversion=off  FilteringAndDerivatives=provide  SimscapeFilterOrder=1  InputFilterTimeConstant=0.001  UdotUserProvided=0
  Solver Configuration : nesl_utility/Solver Configuration  PhysicalDomain=network_engine_domain  SubClassName=solver  LeftPortType=input  RightPortType=generic  Tones=[]  Harmonics=[]  SimulateNoise=off  Profile=off  UseLocalSampling=off  EnableSwitchedLinearOptims=on  FrequencyDomain=off  UseCCode=off  RelTol=0.001  AbsTol=0.001  MinStep=1e-09  ToWorkspace=off  RevertToSquareIcSolve=off  NumHomotopyIterations=100  PhasorMode=off  PhasorModeNumHarmonics=1  ConsistencySolver=NEWTON_XTOL_AFTER_FTOL  IndexReductionMethod=DerivativeReplacement  DoDC=off  ResidualTolerance=1e-09  ConsistencyTolSource=GLOBAL  ConsistencyAbsTol=0.001  ConsistencyRelTol=0.001  ConsistencyTolFactor=0.001  UseLocalSolver=off  LocalSolverChoice=NE_BACKWARD_EULER_ADVANCER  ResolveIndetEquations=on  FunctionEvalNumThread=1  LocalSolverSampleTime=0.001  DoFixedCost=off  MaxNonlinIter=3  MaxModeIter=2  ComputeImpulses=off  ImpulseIterations=2  LinearAlgebra=auto  LinearAlgebraNumThread=0  EquationFormulation=NE_TIME_EF  DelaysMemoryBudget=1024  AutomaticFiltering=on  FilteringTimeConstant=0.001  PartitionStorageMethod=AS_NEEDED  PartitionMemoryBudget=1024  PartitionMethod=ROBUST  MultibodyUseLocalSolver=off  MultibodyLocalSolverChoice=ODE1  MultibodyLocalSolverSampleTime=0.001
  omega_N1 : Outport
  theta_N1 : Outport  Port=2
  wires:
  PS-Simulink Converter1/1 -> theta_N1/1
  PS-Simulink Converter/1 -> omega_N1/1
  Torque_LPT/1 -> Simulink-PS Converter/1
  Torque_Load/1 -> Gain/1
  Gain/1 -> Simulink-PS Converter1/1
  connections:
  Ideal Rotational Motion Sensor/RConn1 -- Ideal Torque Source/LConn1 -- Ideal Torque Source1/LConn1 -- Solver Configuration/RConn1 -- Mechanical Rotational Reference/LConn1
  Rotational Damper/RConn1 -- Ideal Rotational Motion Sensor/LConn1
  Inertia/RConn1 -- Rotational Damper/LConn1
  PS-Simulink Converter/LConn1 -- Ideal Rotational Motion Sensor/RConn2
  PS-Simulink Converter1/LConn1 -- Ideal Rotational Motion Sensor/RConn3
  Simulink-PS Converter1/RConn1 -- Ideal Torque Source1/RConn1
  Simulink-PS Converter/RConn1 -- Ideal Torque Source/RConn1
  Ideal Torque Source/RConn2 -- Ideal Torque Source1/RConn2 -- Inertia/LConn1

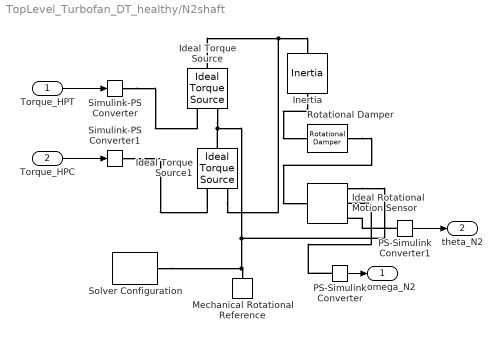
== system TopLevel_Turbofan_DT_healthy/N2shaft ==
  Torque_HPT : Inport
  Torque_HPC : Inport  Port=2
  Ideal Rotational Motion Sensor : fl_lib/Mechanical/Mechanical Sensors/Ideal Rotational Motion Sensor  reference=foundation.enum.MeasurementReference.difference  acceleration_port=false  velocity_port=true  position_port=true  wrap_angle=false  offset=0 rad
  Ideal Torque Source : fl_lib/Mechanical/Mechanical Sources/Ideal Torque Source
  Ideal Torque Source1 : fl_lib/Mechanical/Mechanical Sources/Ideal Torque Source
  Inertia : fl_lib/Mechanical/Rotational Elements/Inertia  inertia=2 kg*m^2  num_ports=foundation.enum.numPorts2.two  w_specify=on  w_priority=High  w=52.36 rad/s  w_nominal_specify=off  w_nominal_value=1  w_nominal_unit=rad/s  t_specify=off  t_priority=None  t=0 N*m  t_nominal_specify=off  t_nominal_value=1  t_nominal_unit=N*m
      settings: InternalSimscapePortConfiguration="{\"Bottom\":[],\"Left\":[{\"id\":\"I\",\"label\":\"\",\"type\":\"foundation.mechanical.rotational.rotational\"}],\"Right\":[{\"id\":\"J\",\"label\":\"\",\"type\":\"foundation.mechanical.rotational.rotational\"}],\"Top\":[]}"
  Mechanical Rotational Reference : fl_lib/Mechanical/Rotational Elements/Mechanical Rotational Reference
  PS-Simulink Converter : nesl_utility/PS-Simulink Converter  PhysicalDomain=network_engine_domain  SubClassName=ps_output  LeftPortType=input  RightPortType=output  PseudoPeriodic=off  Frequencies=[]  VectorFormat=inherit  Unit=rad/s  AffineConversion=off
  PS-Simulink Converter1 : nesl_utility/PS-Simulink Converter  PhysicalDomain=network_engine_domain  SubClassName=ps_output  LeftPortType=input  RightPortType=output  PseudoPeriodic=off  Frequencies=[]  VectorFormat=inherit  Unit=rad  AffineConversion=off
  Rotational Damper : sdl_lib/Couplings & Drives/Springs & Dampers/Rotational Damper  D=1 N*m*s/rad  thermal_port=simscape.enum.thermaleffects.omit  thermal_mass=50 kJ/K  temperature_specify=off  temperature_priority=High  temperature=300 K  temperature_nominal_specify=off  temperature_nominal_value=1  temperature_nominal_unit=K
  Simulink-PS Converter : nesl_utility/Simulink-PS Converter  PhysicalDomain=network_engine_domain  SubClassName=ps_input  LeftPortType=input  RightPortType=output  PseudoPeriodic=off  Frequencies=[]  NoiseDistribution=none  NoiseParameters=[]  Unit=N*m  AffineConversion=off  FilteringAndDerivatives=provide  SimscapeFilterOrder=1  InputFilterTimeConstant=0.001  UdotUserProvided=0
  Simulink-PS Converter1 : nesl_utility/Simulink-PS Converter  PhysicalDomain=network_engine_domain  SubClassName=ps_input  LeftPortType=input  RightPortType=output  PseudoPeriodic=off  Frequencies=[]  NoiseDistribution=none  NoiseParameters=[]  Unit=N*m  AffineConversion=off  FilteringAndDerivatives=provide  SimscapeFilterOrder=1  InputFilterTimeConstant=0.001  UdotUserProvided=0
  Solver Configuration : nesl_utility/Solver Configuration  PhysicalDomain=network_engine_domain  SubClassName=solver  LeftPortType=input  RightPortType=generic  Tones=[]  Harmonics=[]  SimulateNoise=off  Profile=off  UseLocalSampling=off  EnableSwitchedLinearOptims=on  FrequencyDomain=off  UseCCode=off  RelTol=0.001  AbsTol=0.001  MinStep=1e-09  ToWorkspace=off  RevertToSquareIcSolve=off  NumHomotopyIterations=100  PhasorMode=off  PhasorModeNumHarmonics=1  ConsistencySolver=NEWTON_XTOL_AFTER_FTOL  IndexReductionMethod=DerivativeReplacement  DoDC=off  ResidualTolerance=1e-09  ConsistencyTolSource=GLOBAL  ConsistencyAbsTol=0.001  ConsistencyRelTol=0.001  ConsistencyTolFactor=0.001  UseLocalSolver=off  LocalSolverChoice=NE_BACKWARD_EULER_ADVANCER  ResolveIndetEquations=on  FunctionEvalNumThread=1  LocalSolverSampleTime=0.001  DoFixedCost=off  MaxNonlinIter=3  MaxModeIter=2  ComputeImpulses=off  ImpulseIterations=2  LinearAlgebra=auto  LinearAlgebraNumThread=0  EquationFormulation=NE_TIME_EF  DelaysMemoryBudget=1024  AutomaticFiltering=on  FilteringTimeConstant=0.001  PartitionStorageMethod=AS_NEEDED  PartitionMemoryBudget=1024  PartitionMethod=ROBUST  MultibodyUseLocalSolver=off  MultibodyLocalSolverChoice=ODE1  MultibodyLocalSolverSampleTime=0.001
  omega_N2 : Outport
  theta_N2 : Outport  Port=2
  wires:
  Torque_HPC/1 -> Simulink-PS Converter1/1
  PS-Simulink Converter1/1 -> theta_N2/1
  Torque_HPT/1 -> Simulink-PS Converter/1
  PS-Simulink Converter/1 -> omega_N2/1
  connections:
  Solver Configuration/RConn1 -- Mechanical Rotational Reference/LConn1 -- Ideal Torque Source/RConn2 -- Ideal Torque Source1/LConn1 -- Ideal Rotational Motion Sensor/RConn1
  Ideal Torque Source/LConn1 -- Ideal Torque Source1/RConn2 -- Inertia/LConn1
  PS-Simulink Converter/LConn1 -- Ideal Rotational Motion Sensor/RConn2
  Simulink-PS Converter1/RConn1 -- Ideal Torque Source1/RConn1
  Simulink-PS Converter/RConn1 -- Ideal Torque Source/RConn1
  PS-Simulink Converter1/LConn1 -- Ideal Rotational Motion Sensor/RConn3
  Inertia/RConn1 -- Rotational Damper/LConn1
  Rotational Damper/RConn1 -- Ideal Rotational Motion Sensor/LConn1

== matlab function TopLevel_Turbofan_DT_healthy/HPC/CorrectedFlow ==
  data: P1 input; Wc output; T1 input
function Wc = Calc_Wc(P1, T1)
% Computes corrected mass flow [kg/s] from inlet total pressure and temperature

    % Constants
    Tref = 288.15;      % Reference temperature [K]
    Pref = 101325;      % Reference pressure [Pa]
    R = 287;            % J/(kg·K), gas constant for air
    A = 0.05;           % Inlet area [m^2]
    V = 100;            % Inlet velocity [m/s]

    % Safe Inputs
    T_safe = max(T1, eps);   % Avoid division by 0
    P_safe = max(P1, eps);   % Avoid division by 0

    % 1. Air density at inlet
    rho = P_safe / (R * T_safe);   % [kg/m^3]

    % 2. Actual mass flow
    m_dot = rho * A * V;           % [kg/s]

    % 3. Corrected mass flow
    temp_ratio = max(T_safe / Tref, eps);
    press_ratio = max(Pref / P_safe, eps);
    Wc = m_dot / sqrt(temp_ratio) * press_ratio;
end

== matlab function TopLevel_Turbofan_DT_healthy/HPC/HPC_Calculations ==
  data: P1 input; P2 output; T1 input; PR input; eta input; N2 input; T2 output; Torque_HPC output; Wc input
function [P2, T2, Torque_HPC] = HPC_CoreCalc(P1, T1, PR, eta, N2, Wc)
% Computes outlet pressure, temperature, and shaft torque for HPC
% Fully protected version for Simulink/Simscape compatibility

    % Constants
    gamma = 1.4;
    cp = 1004;
    Tref = 288.15;
    Pref = 101325;

    % Clamp all critical inputs to safe non-zero minimums
    P1_safe = max(P1, eps);
    T1_safe = max(T1, eps);
    PR_safe = max(PR, eps);
    eta_safe = max(eta, eps);
    omega = max(N2 * 2 * pi / 60, eps);  % rad/s

    % 1) Outlet pressure
    P2 = P1_safe * PR_safe;

    % 2) Outlet temperature using isentropic relation with efficiency
    T2 = T1_safe * (1 + (1 / eta_safe) * (PR_safe^((gamma - 1) / gamma) - 1));

    % 3) Actual mass flow from corrected flow
    temp_ratio = max(T1_safe / Tref, eps);
    press_ratio = max(P1_safe / Pref, eps);
    m_dot = Wc * sqrt(temp_ratio) * press_ratio;

    % 4) Enthalpy rise
    delta_h = cp * (T2 - T1_safe);

    % 5) Torque on N2 shaft
    torque_raw = (m_dot * delta_h) / omega;

    % 6) Final torque clamp to avoid inf/nan
    Torque_HPC = min(max(torque_raw, -1e6), 1e6);
end

== matlab function TopLevel_Turbofan_DT_healthy/FanNozzle/ComputeCoreThrust ==
  data: T1_fan input; Thrust output; m_dot_bypass input
function Thrust = ComputeFanThrust(T1_fan, m_dot_bypass)
    cp = 1004;             % J/kg·K (air)
    T_ambient = 288;       % K
    V_ambient = 0;         % m/s, stationary aircraft

    if T1_fan > T_ambient
        V_exit = sqrt(2 * cp * (T1_fan - T_ambient));
    else
        V_exit = 0;
    end

    Thrust = m_dot_bypass * (V_exit - V_ambient);
end

== matlab function TopLevel_Turbofan_DT_healthy/CoreNozzle/ComputeCoreThrust ==
  data: T7_in input; Thrust output; m_dot_core input
function Thrust = ComputeCoreThrust(T7_in, m_dot_core)
    cp = 1150;           % J/kg·K (core gas specific heat)
    T_ambient = 288;     % K (standard sea level)
    V_ambient = 0;       % m/s (static case)
    
    % Ensure physical realism
    if T7_in > T_ambient
        V_exit = sqrt(2 * cp * (T7_in - T_ambient));
    else
        V_exit = 0;
    end

    Thrust = m_dot_core * (V_exit - V_ambient);
end

== matlab function TopLevel_Turbofan_DT_healthy/FMS1/AtmosphereModel ==
  data: Altitude input; P0 output; T0 output
function [P0, T0] = AtmosphereModel(Altitude)
% Calculates ambient pressure (P0) and temperature (T0) using ISA model

    T0_sea = 288.15;   % Sea level temperature (K)
    P0_sea = 101325;   % Sea level pressure (Pa)
    L = 0.0065;        % Lapse rate (K/m)
    R = 287.05;        % Gas constant (J/kg·K)
    g = 9.80665;       % Gravity (m/s²)

    if Altitude < 11000
        T0 = T0_sea - L * Altitude;
        P0 = P0_sea * (1 - (L * Altitude) / T0_sea)^(g / (R * L));
    else
        T0 = 216.65;
        P11 = P0_sea * (1 - (L * 11000) / T0_sea)^(g / (R * L));
        P0 = P11 * exp(-g * (Altitude - 11000) / (R * T0));
    end
end

== matlab function TopLevel_Turbofan_DT_healthy/Fan/Fan_CoreCalc ==
  data: P0_fan input; P1_fan output; T0_fan input; PR input; eta_fan input; N1 input; Wc_total input; BPR input; T1_fan_raw output; Torque_fan output; Wc_core output; m_dot_core output
function [P1_fan, T1_fan_raw, Torque_fan, Wc_core, m_dot_core] = Fan_CoreCalc( ...
          P0_fan, T0_fan, PR, eta_fan, N1, Wc_total, BPR)
% Master-level fan thermodynamics and torque with full guards

    % === CONSTANTS ===
    gamma = 1.4;
    cp = 1004;              % [J/(kg·K)]
    Tref = 288.15;          % [K]
    Pref = 101325;          % [Pa]

    % === INPUT SANITY GUARDS ===
    PR       = min(max(PR, 1.01), 2.5);        % Typical fan PR: 1.2–2.0
    eta_fan  = min(max(eta_fan, 0.3), 0.98);   % Reasonable range
    N1       = max(N1, 1e-3);                  % RPM ≥ 0.001
    P0_fan   = max(P0_fan, 50000);             % Prevent vacuum
    T0_fan   = max(T0_fan, 200);               % Prevent < -70°C
    Wc_total = max(Wc_total, 1e-3);            % ≥ 1 g/s
    BPR      = max(BPR, 0);                    % ≥ 0

    % === 1. Outlet Pressure ===
    P1_fan = P0_fan * PR;

    % === 2. Outlet Temperature ===
    T1_fan_raw = T0_fan * (1 + (1 / eta_fan) * (PR^((gamma - 1)/gamma) - 1));

    % === 3. Angular velocity (rad/s) ===
    omega1 = N1 * 2 * pi / 60;

    % === 4. Actual mass flow from corrected ===
    temp_ratio  = max(T0_fan / Tref, eps);
    press_ratio = max(P0_fan / Pref, eps);
    m_dot_total = Wc_total * sqrt(temp_ratio) * press_ratio;

    % === 5. Core vs bypass flow ===
    m_dot_core = m_dot_total / (1 + BPR);

    % === 6. Output corrected core flow ===
    Wc_core = m_dot_core / sqrt(temp_ratio) * (Pref / P0_fan);

    % === 7. Enthalpy rise ===
    delta_T = max(T1_fan_raw - T0_fan, 0);   % Prevent negative ΔT
    delta_h = cp * delta_T;

    % === 8. Torque calculation ===
    raw_torque = (m_dot_total * delta_h) / omega1;

    % === 9. Clamp torque to safe range ===
    Torque_fan = min(max(raw_torque, -1e6), 1e6);  % ±1 MN·m max

    % === Optional Debug Print ===
    % fprintf('[FAN] N1 = %.2f RPM, PR = %.2f, η = %.2f, Torque = %.2f\n', ...
    %         N1, PR, eta_fan, Torque_fan);
end

== matlab function TopLevel_Turbofan_DT_healthy/Fan/Calc_Fan_Wc ==
  data: P0_fan input; Wc_total output; T0_fan input
function Wc_total = Calc_Fan_Wc(P0_fan, T0_fan)
% Return corrected total mass-flow (core + bypass) in kg/s.
% Fully guarded for Simulink/Simscape code-gen.

    % ----- constants ----------------------------------------------------
    Tref = 288.15;          % K
    Pref = 101325;          % Pa
    R    = 287;             % J/(kg·K)
    A    = 0.50;            % m^2   (fan face area)
    V    = 120;             % m/s   (inlet velocity estimate)

    % ----- protect inputs ----------------------------------------------
    P  = max(P0_fan,  1e-3);    % avoid /0
    T  = max(T0_fan,  1e-3);

    % ----- density & actual mass-flow ----------------------------------
    rho          = P / (R * T);               % kg/m^3
    m_dot_total  = rho * A * V;               % kg/s

    % ----- corrected flow ----------------------------------------------
    temp_ratio   = max(T / Tref, eps);
    press_ratio  = max(Pref / P, eps);
    Wc_total_raw = m_dot_total / sqrt(temp_ratio) * press_ratio;

    % ----- clamp to physically plausible range -------------------------
    Wc_total = min(max(Wc_total_raw, 10), 2000);   % kg/s
end

== matlab function TopLevel_Turbofan_DT_healthy/LPT/MATLAB Function ==
  data: P6_in input; T6_in input; P7_out output; PR_LPT input; eta_LPT input; N1_RPM input; T7_out output; Torque_LPT output; m_dot_core input
function [P7_out, T7_out, Torque_LPT] = ...
    LPT_CalcCore(P6_in, T6_in, PR_LPT, eta_LPT, N1_RPM, m_dot_core)

% ===== constants & guards ==============================================
gamma = 1.4;  cp = 1004;

P6  = max(P6_in,  1e-3);
T6  = max(T6_in,  1e-3);
PR  = max(min(PR_LPT,0.98),0.50);    % turbine PR ≤ 1
eta = max(eta_LPT, 1e-3);
rpm = max(N1_RPM,  1e-3);
md  = max(m_dot_core, 1e-3);

% ===== outlet P/T =======================================================
P7_out = P6 * PR;
T7_out = T6 * (1 - eta*(1 - PR^((gamma-1)/gamma)));

% ===== torque ===========================================================
omega      = rpm * 2*pi/60;            % rad/s
delta_h    = cp * max(T6 - T7_out, 0); % positive J/kg
torque_raw = (md * delta_h) / max(omega, eps);
Torque_LPT = torque_raw;
end

== matlab function TopLevel_Turbofan_DT_healthy/LPC/LPC_CoreCalc ==
  data: P2_in input; P3 output; T2_in input; PR_LPC input; eta_LPC input; N1_RPM input; Wc_core_in input; T3 output; Torque_LPC output; m_dot_core output
function [P3, T3, Torque_LPC, m_dot_core] = ...
    LPC_CoreCalc(P2_in, T2_in, PR_LPC, eta_LPC, N1_RPM, Wc_core_in)

% ===== constants & guards ==============================================
gamma = 1.4;  cp = 1004;  Tref = 288.15;  Pref = 101325;

P2 = max(P2_in,    1e-3);
T2 = max(T2_in,    1e-3);
PR = max(PR_LPC,   1.0);      % compressor PR ≥ 1
eta = max(eta_LPC, 1e-3);
rpm = max(N1_RPM,  1e-3);
Wc  = max(Wc_core_in, 1e-3);

% ===== outlet P/T =======================================================
P3 = P2 * PR;
T3 = T2 * (1 + (1/eta)*(PR^((gamma-1)/gamma) - 1));

% ===== mass-flow recovery (real kg/s) ===================================
temp_ratio  = max(T2 / Tref, eps);
press_ratio = max(P2 / Pref, eps);
m_dot_core  = Wc * sqrt(temp_ratio) * press_ratio;

% ===== torque ===========================================================
omega  = max(rpm * 2*pi/60, eps);
delta_h = cp * max(T3 - T2, 0);
torque_raw = (m_dot_core * delta_h) / omega;
Torque_LPC = min(max(torque_raw, -1e6), 1e6);
end

== matlab function TopLevel_Turbofan_DT_healthy/HPT/ComputeTorqueFinal ==
  data: thermoTorque input; Torque_HPT output; mapTorque input
function Torque_HPT = ComputeTorqueFinal(thermoTorque, mapTorque)
    % Combine both torque calculations with 50/50 weighting
    Torque_HPT = 0.5 * thermoTorque + 0.5 * mapTorque;
end

== matlab function TopLevel_Turbofan_DT_healthy/HPT/HPT_TempCalc ==
  data: P5_in input; P6_out output; T5_in input; Eff_HPT input; T6_out output
function [P6_out, T6_out] = HPT_TempCalc(P5_in, T5_in, Eff_HPT)
    gamma = 1.33;
    PR_turb = 1.0;  % Assume isobaric turbine
    T6_ideal = T5_in * (PR_turb)^((gamma-1)/gamma);
    T6_out = T5_in - Eff_HPT * (T5_in - T6_ideal);
    P6_out = P5_in;  % no pressure drop assumption
end

== matlab function TopLevel_Turbofan_DT_healthy/HPT/HPT_TorqueCalc ==
  data: m_dot5 input; Torque_HPT output; T5_in input; T6_out input; omega_N2 input
function Torque_HPT = HPT_TorqueCalc(m_dot5, T5_in, T6_out, omega_N2)
    cp = 1150;  % J/kg-K
    work = cp * (T5_in - T6_out);

    % Safety wrappers
    omega_safe = max(omega_N2, eps);
    m_dot_safe = max(m_dot5, eps);      % protect m_dot
    work_safe = max(work, 0);           % assume zero torque if temp reversed

    Torque_HPT = (m_dot_safe * work_safe) / omega_safe;
end
